simulink model "BuckConverter_Speed_first"  (R2021a)
settings: Solver=ode15s  StartTime=0.0  StopTime=0.01  MaxStep=1/(4*fsw)  RelTol=1e-3
PreLoadFcn:
  | Param_BuckConvertrer
undefined symbols (not defined in the file): DeadTime, fsw, MaxDuty, MinDuty, TimerCountMax
libraries: fl_lib x10, nesl_utility x6, ee_lib x2, eeGeneralControl x1, simulink x1
settings Model: Creator=ykamatan  LastModifiedBy=ykamatan
settings SimscapeCC: SimscapeLogType=local  SimscapeLogSimulationStatistics=on  SimscapeLogName=simlogBuckConverter  SimscapeLogLimitData=off

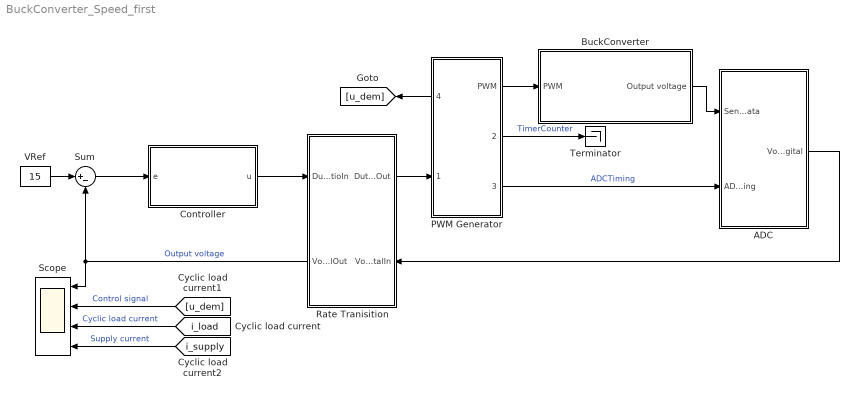
== system BuckConverter_Speed_first ==
  ADC : Subsystem
      settings: PortSchema="{\"entries\":[{\"content\":{\"sides\":[{\"content\":{\"connectorIds\":[]},\"type\":\"ConnectorPlacement.EquallySpacedRectSide\",\"uuid\":\"bf6494ef-7686-469c-b9a7-d936a514d7bb\"},{\"content\":{\"connectorIds\":[],\"side\":\"RIGHT\"},\"type\":\"ConnectorPlacement.EquallySpacedRectSide\",\"uuid\":\"0950a60e-c0cc-4272-a83f-094f77322897\"},{\"content\":{\"connectorIds\":[\"In1\",\"In2\"],\"side\":\"TOP\"},\"type\":\"ConnectorPlacement.EquallySpacedRectSide\",\"uuid\":\"00c09912-fdc2-48e7-8c4d-a5acc3c27a79\"},{\"content\":{\"connectorIds\":[\"Out1\"],\"side\":\"BOTTOM\"},\"type\":\"ConnectorPlacement.EquallySpacedRectSide\",\"uuid\":\"03f25cec-c069-475d-9cdb-f76905a62459\"}]},\"type\":\"ConnectorPlacement.EquallySpacedConnector\",\"uuid\":\"810e678a-0254-41ea-a955-7b792bb7817f\"}],\"packageUris\":[\"http://schema.mathworks.com/mf0/Connector/R2020b\"],\"version\":\"1.0\"}"
  BuckConverter : Subsystem
  Controller : Subsystem  Variant=on  VariantControlMode=label  LabelModeActiveChoice=Discrete
      settings: AttributesFormatString=%<BlockChoice>  PortSchema="{\"entries\":[{\"content\":{\"sides\":[{\"content\":{\"connectorIds\":[\"Out1\"]},\"type\":\"ConnectorPlacement.EquallySpacedRectSide\",\"uuid\":\"685b2dc6-4f02-4a7b-a6bf-88e3d36bc83e\"},{\"content\":{\"connectorIds\":[\"In1\"],\"side\":\"RIGHT\"},\"type\":\"ConnectorPlacement.EquallySpacedRectSide\",\"uuid\":\"22f020c9-8565-4c84-885b-1a26e9339655\"},{\"content\":{\"connectorIds\":[],\"side\":\"TOP\"},\"type\":\"ConnectorPlacement.EquallySpacedRectSide\",\"uuid\":\"adb99d42-7d64-4d3d-be76-0d683fbfb3ea\"}]},\"type\":\"ConnectorPlacement.EquallySpacedConnector\",\"uuid\":\"e1039069-23fc-4515-974b-2f79b4645018\"}],\"packageUris\":[\"http://schema.mathworks.com/mf0/Connector/R2020b\"],\"version\":\"1.0\"}"
  PWM Generator : Subsystem
      settings: PortSchema="{\"entries\":[{\"content\":{\"sides\":[{\"content\":{\"connectorIds\":[\"Out4\",\"In1\"]},\"type\":\"ConnectorPlacement.EquallySpacedRectSide\",\"uuid\":\"f1ce74a1-1a8f-47f7-9cd0-3fde2298587e\"},{\"content\":{\"connectorIds\":[\"Out1\",\"Out2\",\"Out3\"],\"side\":\"RIGHT\"},\"type\":\"ConnectorPlacement.EquallySpacedRectSide\",\"uuid\":\"07a21a0a-7c65-47ad-a570-3864e55861a7\"},{\"content\":{\"connectorIds\":[],\"side\":\"TOP\"},\"type\":\"ConnectorPlacement.EquallySpacedRectSide\",\"uuid\":\"8095ad0e-75cb-4fce-a461-a34c62050671\"},{\"content\":{\"connectorIds\":[],\"side\":\"BOTTOM\"},\"type\":\"ConnectorPlacement.EquallySpacedRectSide\",\"uuid\":\"dd227050-6090-4f15-8849-81744ca66faf\"}]},\"type\":\"ConnectorPlacement.EquallySpacedConnector\",\"uuid\":\"2f82d847-9a80-4fd2-b8a2-8a906b7e656c\"}],\"packageUris\":[\"http://schema.mathworks.com/mf0/Connector/R2020b\"],\"version\":\"1.0\"}"
  "Rate Tranisition " : Subsystem
      settings: PortSchema="{\"entries\":[{\"content\":{\"sides\":[{\"content\":{\"connectorIds\":[\"In1\",\"Out2\"]},\"type\":\"ConnectorPlacement.EquallySpacedRectSide\",\"uuid\":\"82fdd683-de0b-47f1-9418-2e57132da0d0\"},{\"content\":{\"connectorIds\":[\"Out1\",\"In2\"],\"side\":\"RIGHT\"},\"type\":\"ConnectorPlacement.EquallySpacedRectSide\",\"uuid\":\"07812756-bbdf-4a3e-b825-c2cce10242a3\"},{\"content\":{\"connectorIds\":[],\"side\":\"TOP\"},\"type\":\"ConnectorPlacement.EquallySpacedRectSide\",\"uuid\":\"2a69d2b0-ad53-492d-9041-fc24e9d8466e\"}]},\"type\":\"ConnectorPlacement.EquallySpacedConnector\",\"uuid\":\"5e8493d4-adb1-45a0-b631-53482b8c22b1\"}],\"packageUris\":[\"http://schema.mathworks.com/mf0/Connector/R2020b\"],\"version\":\"1.0\"}"
  Scope : Scope  NumInputPorts=4
  Sum : Sum  Inputs=|+-  InputSameDT=on  SaturateOnIntegerOverflow=on  OutDataTypeStr=Inherit: Same as first input
  Terminator : Terminator
  VRef : Constant  Value=15
  wires:
  Controller/1(u) -> "Rate Tranisition "/1(DutyRatioIn)
  Sum/1 -> Controller/1(e)
  VRef/1 -> Sum/1
  PWM Generator/3(TopDetect) -> ADC/2(ADCTiming)  "ADCTiming"
  [u_dem] -> Scope/2  "Control signal"
  [i_load] -> Scope/3  "Cyclic load current"
  [i_supply] -> Scope/4  "Supply current"
  ADC/1(Vo_Digital) -> "Rate Tranisition "/2(Vo_DigitalIn)
  "Rate Tranisition "/2(Vo_DigitalOut) -> Sum/2, Scope/1  "Output voltage"
  "Rate Tranisition "/1(DutyRatioOut) -> PWM Generator/1(DutyRatio)
  PWM Generator/4(DutyRatio_limited) -> [u_dem]
  PWM Generator/1(PWM) -> BuckConverter/1(PWM)
  BuckConverter/1(Output voltage) -> ADC/1(SensorData)
  PWM Generator/2(TimerCounter) -> Terminator/1  "TimerCounter"

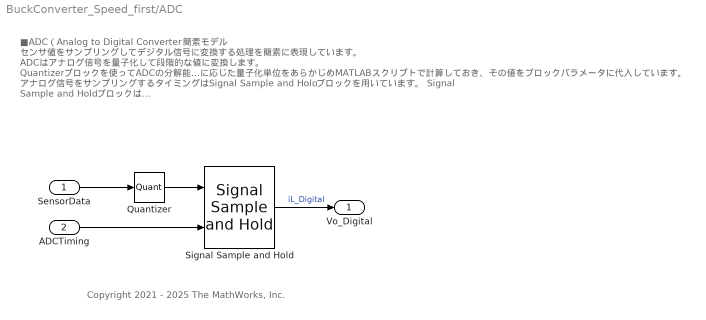
== system BuckConverter_Speed_first/ADC ==
  note: ■ADC（Analog to Digital Converter)簡素モデル
      | センサ値をサンプリングしてデジタル信号に変換する処理を簡素に表現しています。
      | ADCはアナログ信号を量子化して段階的な値に変換します。
      | Quantizerブロックを使ってADCの分解能に応じた量子化単位をあらかじめMATLABスクリプトで計算しておき、その値をブロックパラメータに代入しています。
      | アナログ信号をサンプリングするタイミングはSignal Sample and Holdブロックを用いています。
      | Signal Sample and Holdブロックは
      | Inにサンプリングしたい信号、Sにサンプリングタイミングを指定するパルス信号を入力することで、
      | そのタイミングでInの値をサンプリングし、それ以降次のパルスが入るまで値を保持します。
  note: Copyright 2021 - 2025 The MathWorks, Inc.
  SensorData : Inport
  ADCTiming : Inport  Port=2
  Quantizer : Quantizer  QuantizationInterval=QuantUnit
  Signal Sample and Hold : eeGeneralControl/Signal Sample and Hold  LabelModeActiveChoice=Discrete  x0=0  Ts=-1
      settings: SourceProductBaseCode=PS
  Vo_Digital : Outport
  wires:
  Quantizer/1 -> Signal Sample and Hold/1
  Signal Sample and Hold/1 -> Vo_Digital/1  "iL_Digital"
  ADCTiming/1 -> Signal Sample and Hold/2
  SensorData/1 -> Quantizer/1

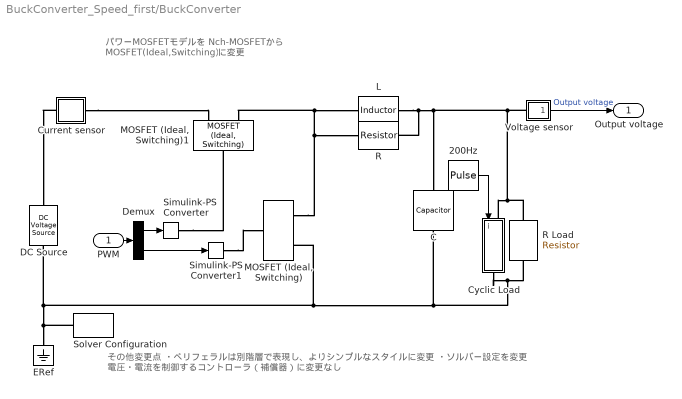
== system BuckConverter_Speed_first/BuckConverter ==
  note: その他変更点
      | ・ペリフェラルは別階層で表現し、よりシンプルなスタイルに変更
      | ・ソルバー設定を変更
      |
      | 電圧・電流を制御するコントローラ（補償器）に変更なし
  note: パワーMOSFETモデルを
      | Nch-MOSFETから
      | MOSFET(Ideal,Switching)に変更
  PWM : Inport
  " C" : fl_lib/Electrical/Electrical Elements/Capacitor  c=22 uF  r=0 Ohm  g=0 1/Ohm  i_specify=off  i_priority=High  i=0 A  i_nominal_specify=off  i_nominal_unit=A  i_nominal_value=1  v_specify=off  v_priority=High  v=0 V  v_nominal_specify=off  v_nominal_unit=V  v_nominal_value=1  vc_specify=on  vc_priority=High  vc=0 V  vc_nominal_specify=off  vc_nominal_unit=V  vc_nominal_value=1
  200Hz : DiscretePulseGenerator  PulseType=Time based  Period=1/200  PulseWidth=50  PhaseDelay=1/400
  Current sensor : Subsystem
  Cyclic Load : Subsystem
  DC Source : fl_lib/Electrical/Electrical Sources/DC Voltage Source  v0=30 V
      settings: AttributesFormatString=%<v0> %<v0_unit>
  Demux : Demux  Outputs=2
  ERef : fl_lib/Electrical/Electrical Elements/Electrical Reference
  L : fl_lib/Electrical/Electrical Elements/Inductor  l=1e-3 H  r=0 Ohm  g=0 1/Ohm  i_specify=off  i_priority=High  i=0 A  i_nominal_specify=off  i_nominal_unit=A  i_nominal_value=1  v_specify=off  v_priority=High  v=0 V  v_nominal_specify=off  v_nominal_unit=V  v_nominal_value=1  i_L_specify=on  i_L_priority=High  i_L=0 A  i_L_nominal_specify=off  i_L_nominal_unit=A  i_L_nominal_value=1
  "MOSFET (Ideal, Switching)" : ee_lib/Semiconductors & Converters/MOSFET (Ideal, Switching)  Rds=0.1 Ohm  Goff=1e-6 1/Ohm  Vth=2 V  diode_param=2  diode_Vf=0.8 V  diode_Ron=0.001 Ohm  diode_Goff=1e-5 1/Ohm  diode_C=50e-9 F  diode_iRM=-235 A  diode_iF=300 A  diode_idot=-50 A/us  diode_trr_param=1  diode_trr_factor=3  diode_trr=15 us  diode_Qrr=1500 s*uA  thermal_loss_option=ee.enum.converters.thermalLossOption.constantvalues  Von_data=[0, 1.1, 1.3, 1.45, 1.75, 2.25, 2.7; 0, 1, 1.15, 1.35, 1.7, 2.35, 3] V  Eon_data=[0, .29, 1.43, 2.86, 5.71, 13.14, 22.86; 0, .57, 2.63, 5.14, 10.29, 20.57, 30.29] * 1e-3 J  Eoff_data=[0, .21, 1.07, 2.14, 4.29, 9.86, 17.14; 0, .43, 1.97, 3.86, 7.71, 15.43, 22.71] * 1e-3 J  Tj=[298.15, 398.15] K  Iout_data=[0, 10, 50, 100, 200, 400, 600] A  Eon_scalar=22.86e-3 J  Eoff_scalar=17.14e-3 J  Voff=300 V  Iout_scalar=600 A  diodeModelType=ee.enum.converters.diodeModelType.pwl  diode_IfMat=[.07, .12, .19, 1.75, 4.24, 7.32, 11.2; .16, .3, .72, 2.14, 4.02, 6.35, 9.12] A  diode_TjVec=[25, 125] degC  diode_VfVec=[.5, .7, .9, 1.3, 1.7, 2.1, 2.5] V  thermal_network_parameterization=ee.enum.thermalNetworkTopology.external  Rth=[.03, .2] K/W  Rth_Foster=[.03, .2] K/W  thermal_mass_parameterization=ee.enum.thermalNetwork.timeconstant  thermal_mass=[3, 25] J/K  thermal_mass_Foster=[33, 50] J/K  thermal_time_constant=[.1, 5] s  thermal_time_constant_Foster=[1, 10] s  thermal_mass_initial_temperatures=[25, 25] degC  junction_thermal_mass=0.1 J/K  vT_specify=off  vT_priority=None  vT=0 V  vT_nominal_specify=off  vT_nominal_unit=V  vT_nominal_value=1  Qj_specify=off  Qj_priority=None  Qj=0 W  Qj_nominal_specify=off  Qj_nominal_unit=W  Qj_nominal_value=1  junction_temperature_specify=off  junction_temperature_priority=None  junction_temperature=25 degC  junction_temperature_nominal_specify=off  junction_temperature_nominal_unit=degC  junction_temperature_nominal_value=1
  "MOSFET (Ideal, Switching)1" : ee_lib/Semiconductors & Converters/MOSFET (Ideal, Switching)  Rds=0.1 Ohm  Goff=1e-6 1/Ohm  Vth=2 V  diode_param=2  diode_Vf=0.8 V  diode_Ron=0.001 Ohm  diode_Goff=1e-5 1/Ohm  diode_C=50e-9 F  diode_iRM=-235 A  diode_iF=300 A  diode_idot=-50 A/us  diode_trr_param=1  diode_trr_factor=3  diode_trr=15 us  diode_Qrr=1500 s*uA  thermal_loss_option=ee.enum.converters.thermalLossOption.constantvalues  Von_data=[0, 1.1, 1.3, 1.45, 1.75, 2.25, 2.7; 0, 1, 1.15, 1.35, 1.7, 2.35, 3] V  Eon_data=[0, .29, 1.43, 2.86, 5.71, 13.14, 22.86; 0, .57, 2.63, 5.14, 10.29, 20.57, 30.29] * 1e-3 J  Eoff_data=[0, .21, 1.07, 2.14, 4.29, 9.86, 17.14; 0, .43, 1.97, 3.86, 7.71, 15.43, 22.71] * 1e-3 J  Tj=[298.15, 398.15] K  Iout_data=[0, 10, 50, 100, 200, 400, 600] A  Eon_scalar=22.86e-3 J  Eoff_scalar=17.14e-3 J  Voff=300 V  Iout_scalar=600 A  diodeModelType=ee.enum.converters.diodeModelType.pwl  diode_IfMat=[.07, .12, .19, 1.75, 4.24, 7.32, 11.2; .16, .3, .72, 2.14, 4.02, 6.35, 9.12] A  diode_TjVec=[25, 125] degC  diode_VfVec=[.5, .7, .9, 1.3, 1.7, 2.1, 2.5] V  thermal_network_parameterization=ee.enum.thermalNetworkTopology.external  Rth=[.03, .2] K/W  Rth_Foster=[.03, .2] K/W  thermal_mass_parameterization=ee.enum.thermalNetwork.timeconstant  thermal_mass=[3, 25] J/K  thermal_mass_Foster=[33, 50] J/K  thermal_time_constant=[.1, 5] s  thermal_time_constant_Foster=[1, 10] s  thermal_mass_initial_temperatures=[25, 25] degC  junction_thermal_mass=0.1 J/K  vT_specify=off  vT_priority=None  vT=0 V  vT_nominal_specify=off  vT_nominal_unit=V  vT_nominal_value=1  Qj_specify=off  Qj_priority=None  Qj=0 W  Qj_nominal_specify=off  Qj_nominal_unit=W  Qj_nominal_value=1  junction_temperature_specify=off  junction_temperature_priority=None  junction_temperature=25 degC  junction_temperature_nominal_specify=off  junction_temperature_nominal_unit=degC  junction_temperature_nominal_value=1
  R : fl_lib/Electrical/Electrical Elements/Resistor  R=10 kOhm  i_specify=off  i_priority=High  i=0 A  i_nominal_specify=off  i_nominal_unit=A  i_nominal_value=1  v_specify=off  v_priority=High  v=0 V  v_nominal_specify=off  v_nominal_unit=V  v_nominal_value=1
  R Load : fl_lib/Electrical/Electrical Elements/Resistor  R=3.75 Ohm  i_specify=off  i_priority=High  i=0 A  i_nominal_specify=off  i_nominal_unit=A  i_nominal_value=1  v_specify=off  v_priority=High  v=0 V  v_nominal_specify=off  v_nominal_unit=V  v_nominal_value=1
  Simulink-PS Converter : nesl_utility/Simulink-PS Converter  PhysicalDomain=network_engine_domain  SubClassName=ps_input  LeftPortType=input  RightPortType=output  PseudoPeriodic=off  Frequencies=[]  NoiseDistribution=none  NoiseParameters=[]  Unit=1  AffineConversion=off  FilteringAndDerivatives=provide  SimscapeFilterOrder=1  InputFilterTimeConstant=0.001  UdotUserProvided=0
      settings: SourceProductBaseCode=PW,SS
  Simulink-PS Converter1 : nesl_utility/Simulink-PS Converter  PhysicalDomain=network_engine_domain  SubClassName=ps_input  LeftPortType=input  RightPortType=output  PseudoPeriodic=off  Frequencies=[]  NoiseDistribution=none  NoiseParameters=[]  Unit=1  AffineConversion=off  FilteringAndDerivatives=provide  SimscapeFilterOrder=1  InputFilterTimeConstant=0.001  UdotUserProvided=0
      settings: SourceProductBaseCode=PW,SS
  Solver Configuration : nesl_utility/Solver Configuration  PhysicalDomain=network_engine_domain  SubClassName=solver  LeftPortType=input  RightPortType=generic  Tones=[]  Harmonics=[]  SimulateNoise=off  Profile=off  UseLocalSampling=off  EnableSwitchedLinearOptims=on  FrequencyDomain=off  UseCCode=off  RelTol=0.001  AbsTol=1e-06  MinStep=1e-09  ToWorkspace=off  RevertToSquareIcSolve=off  NumHomotopyIterations=100  PhasorMode=off  PhasorModeNumHarmonics=1  DoDC=off  ResidualTolerance=1e-9  UseLocalSolver=off  LocalSolverChoice=NE_BACKWARD_EULER_ADVANCER  LocalSolverSampleTime=1e-7  DoFixedCost=off  MaxNonlinIter=12  MaxModeIter=2  ComputeImpulses=off  ImpulseIterations=1  LinearAlgebra=auto  EquationFormulation=NE_TIME_EF  DelaysMemoryBudget=1024  AutomaticFiltering=on  FilteringTimeConstant=0.001  PartitionStorageMethod=AS_NEEDED  PartitionMemoryBudget=1024  PartitionMethod=FAST
      settings: SourceProductBaseCode=PW,SS
  Voltage sensor : Subsystem
      settings: CopyFcn=set_param(gcb,'LinkStatus','none')
  Output voltage : Outport
  wires:
  Demux/1 -> Simulink-PS Converter/1
  Demux/2 -> Simulink-PS Converter1/1
  PWM/1 -> Demux/1
  200Hz/1 -> Cyclic Load/1(i)
  Voltage sensor/1(v) -> Output voltage/1  "Output voltage"
  connections:
  R Load/LConn1 -- Voltage sensor/LConn1 -- L/LConn1 -- R/LConn1 -- " C"/LConn1 -- Cyclic Load/LConn1
  "MOSFET (Ideal, Switching)"/RConn1 -- R/RConn1 -- L/RConn1 -- "MOSFET (Ideal, Switching)1"/RConn2
  " C"/RConn1 -- Cyclic Load/RConn1 -- R Load/RConn1 -- "MOSFET (Ideal, Switching)"/RConn2 -- DC Source/RConn1 -- Solver Configuration/RConn1 -- ERef/LConn1
  Current sensor/RConn1 -- "MOSFET (Ideal, Switching)1"/RConn1
  Current sensor/LConn1 -- DC Source/LConn1
  Simulink-PS Converter1/RConn1 -- "MOSFET (Ideal, Switching)"/LConn1
  Simulink-PS Converter/RConn1 -- "MOSFET (Ideal, Switching)1"/LConn1

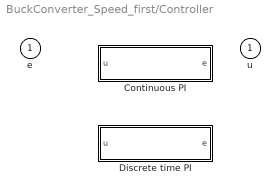
== system BuckConverter_Speed_first/Controller ==
  e : Inport
  Continuous PI : Subsystem  VariantControl=Continuous
  Discrete time PI : Subsystem  VariantControl=Discrete
  u : Outport  VectorParamsAs1DForOutWhenUnconnected=off

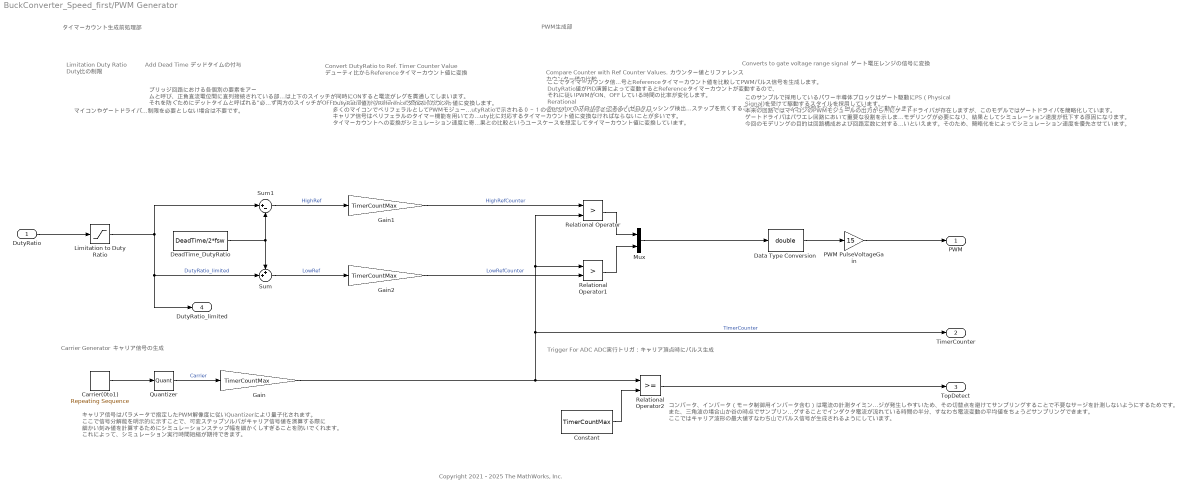
== system BuckConverter_Speed_first/PWM Generator ==
  note: PWM生成部
  note: タイマーカウント生成前処理部
  note: Limitation
      | Duty Ratio
      |
      | Duty比の制限
  note: キャリア信号はパラメータで指定したPWM解像度に従いQuantizerにより量子化されます。
      | ここで信号分解能を明示的に示すことで、可変ステップソルバがキャリア信号値を演算する際に
      | 細かい刻み値を計算するためにシミュレーションステップ幅を細かくしすぎることを防いでくれます。
      | これによって、シミュレーション実行時間短縮が期待できます。
  note: Converts to gate voltage range signal
      | ゲート電圧レンジの信号に変換
  note: Compare Counter with Ref Counter Values.
      | カウンター値とリファレンス カウンター値の比較
  note: Trigger For ADC
      | ADC実行トリガ：キャリア頂点時にパルス生成
  note: Convert DutyRatio to　Ref. Timer Counter Value
      | デューティ比からReferenceタイマーカウント値に変換
  note: Add Dead Time
      | デッドタイムの付与
  note: Carrier Generator
      | キャリア信号の生成
  note: Copyright 2021 - 2025 The MathWorks, Inc.
  note: ブリッジ回路における各個別の要素をアー ムと呼び、正負直流電位間に直列接続されている部分を上下一組でレグと呼びます。今回回路に用いているハーフブリッジ回路は単一のレグに相当します。レグを駆動する際には上下のスイッチが同時にONすると電流がレグを貫通してしまいます。
      | それを防ぐためにデットタイムと呼ばれる”必ず両方のスイッチがOFFとなる時間”を付与することで貫通を防ぎます。
  note: DutyRatio値からReferenceタイマーカウント値に変換します。
      | 多くのマイコンでペリフェラルとしてPWMモジュールが搭載されていますが、DutyRatioで示される０～１の値を使ってPWM波形を生成していません。
      |
      | キャリア信号はペリフェラルのタイマー機能を用いてカウントアップ・カウントダウンによって生成されるカウント値として指定されるので、Duty値もまた、Duty比に対応するタイマーカウント値に変換なければならないことが多いです。
      | タイマーカウントへの変換がシミュレーション速度に寄与する影響度は少ないですが、実機実験でのデバック結果との比較というユースケースを想定してタイマーカウント値に変換しています。
  note: ここでタイマーカウンタ信号とReferenceタイマーカウント値を比較してPWMパルス信号を生成します。
      |
      | DutyRatio値がPID演算によって変動するとReferenceタイマーカウントが変動するので、
      | それに従いPWMがON、OFFしている時間の比率が変化します。
      | Rerational Operatorのプロパティである「ゼロクロッシング検出を有効にする」を有効にすることで、可変ステップソルバは比較によって値が変動するタイミングで細かくステップを刻み、そうでない箇所ではタイムステップを荒くすることでシミュレーション時間をなるべく短くするように動作します。
  note: このサンプルで採用しているパワー半導体ブロックはゲート駆動にPS（Physical Signal)を受けて駆動するスタイルを採用しています。
      |
      | 本来の回路ではマイコンのPWMモジュールの出力からパワー半導体デバイスの間にゲートドライバが存在しますが、このモデルではゲートドライバを簡略化しています。
      |
      | ゲートドライバはパワエレ回路において重要な役割を示しますが、正確な挙動表現には細かいモデリングが必要になり、結果としてシミュレーション速度が低下する原因になります。
      | 今回のモデリングの目的は回路構成および回路定数に対する適切な制御則の導出であるため、目的に対してゲートドライバの詳細表現は影響度が少ないといえます。そのため、簡略化をによってシミュレーション速度を優先させています。
  note: コンバータ、インバータ（モータ制御用インバータ含む）は電流の計測タイミングをPWMキャリア信号と同期させることが多く、ノコギリ波の頂点、もしくは三角波の山か谷のタイミングでADCのサンプリングを行います。これはPWMパルス電圧が切り替わる瞬間は電流サージが発生しやすいため、その切替点を避けてサンプリングすることで不要なサージを計測しないようにするためです。
      | また、三角波の場合山か谷の時点でサンプリングすることでインダクタ電流が流れている時間の半分、すなわち電流変動の平均値をちょうどサンプリングできます。
      | ここではキャリア波形の最大値すなわち山でパルス信号が生成されるようにしています。
  note: マイコンやゲートドライバ、制御ICにはDutyの最大値、最小値が指定されているものも多いためここで制限を設けています。制限を必要としない場合は不要です。
  DutyRatio : Inport
  Carrier(0to1) : simulink/Sources/Repeating Sequence  rep_seq_t=[0 1/fsw/2 1/fsw]  rep_seq_y=[1 0 1]
  Constant : Constant  Value=TimerCountMax  OutDataTypeStr=uint16
  Data Type Conversion : DataTypeConversion  OutDataTypeStr=double
  DeadTime_DutyRatio : Constant  Value=DeadTime/2*fsw  OutDataTypeStr=double
  Gain : Gain  Gain=TimerCountMax  OutDataTypeStr=double
  Gain1 : Gain  Gain=TimerCountMax
  Gain2 : Gain  Gain=TimerCountMax  OutDataTypeStr=double
  Limitation to Duty Ratio : Saturate  UpperLimit=MaxDuty  LowerLimit=MinDuty
  Mux : Mux  Inputs=2
  PWM PulseVoltageGain : Gain  Gain=15
  Quantizer : Quantizer  QuantizationInterval=PWM_Resolution
  Relational Operator : RelationalOperator  Operator=>  OutDataTypeStr=boolean  RndMeth=Simplest  InputSameDT=on
  Relational Operator1 : RelationalOperator  Operator=>  OutDataTypeStr=boolean  RndMeth=Simplest  InputSameDT=on
  Relational Operator2 : RelationalOperator  OutDataTypeStr=boolean  RndMeth=Simplest
  Sum : Sum  Inputs=++|
  Sum1 : Sum  Inputs=|+-
  PWM : Outport
  TimerCounter : Outport  Port=2
  TopDetect : Outport  Port=3
  DutyRatio_limited : Outport  Port=4
  wires:
  Relational Operator1/1 -> Mux/2
  Data Type Conversion/1 -> PWM PulseVoltageGain/1
  Mux/1 -> Data Type Conversion/1
  Relational Operator/1 -> Mux/1
  DutyRatio/1 -> Limitation to Duty Ratio/1
  PWM PulseVoltageGain/1 -> PWM/1
  Carrier(0to1)/1 -> Quantizer/1
  Sum/1 -> Gain2/1  "LowRef"
  Limitation to Duty Ratio/1 -> DutyRatio_limited/1, Sum/2, Sum1/1  "DutyRatio_limited"
  DeadTime_DutyRatio/1 -> Sum1/2, Sum/1
  Constant/1 -> Relational Operator2/2
  Relational Operator2/1 -> TopDetect/1
  Quantizer/1 -> Gain/1  "Carrier"
  Gain/1 -> Relational Operator2/1, Relational Operator1/1, Relational Operator/2, TimerCounter/1  "TimerCounter"
  Gain1/1 -> Relational Operator/1  "HighRefCounter"
  Sum1/1 -> Gain1/1  "HighRef"
  Gain2/1 -> Relational Operator1/2  "LowRefCounter"

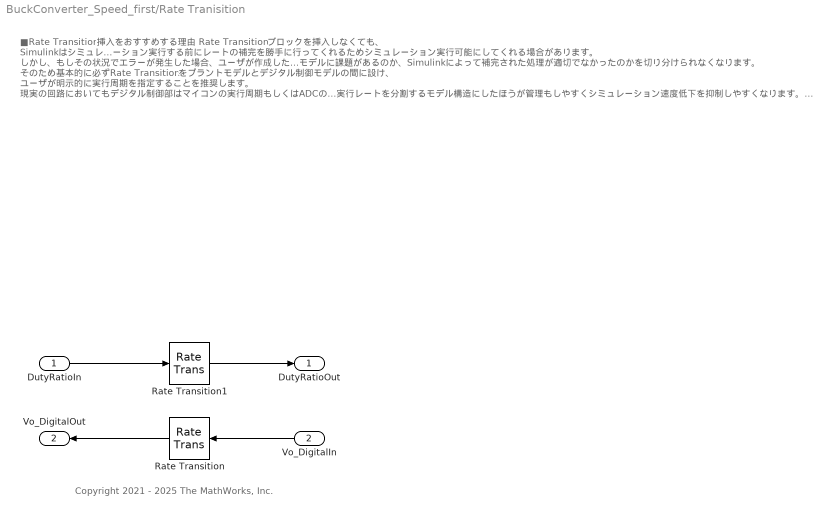
== system BuckConverter_Speed_first/Rate Tranisition  ==
  note: ■Rate Transition挿入をおすすめする理由
      | Rate Transitionブロックを挿入しなくても、
      | Simulinkはシミュレーション実行する前にレートの補完を勝手に行ってくれるためシミュレーション実行可能にしてくれる場合があります。
      |
      | しかし、もしその状況でエラーが発生した場合、ユーザが作成したモデルに課題があるのか、Simulinkによって補完された処理が適切でなかったのかを切り分けられなくなります。
      |
      | そのため基本的に必ずRate Transitionをプラントモデルとデジタル制御モデルの間に設け、
      | ユーザが明示的に実行周期を指定することを推奨します。
      |
      | 現実の回路においてもデジタル制御部はマイコンの実行周期もしくはADCの変換タイミングをトリガーに周期的に処理を行うため、明示的に実行レートを分割するモデル構造にしたほうが管理もしやすくシミュレーション速度低下を抑制しやすくなります。
      |
      | ■Rate Transitionのブロックパラメータ設定方法
      | ・データ転送中の整合性を確保
      | ・確定的にデータ転送を確保（最大遅延）
      | のチェックを入れておくことで、想定される最大のサンプリング遅れでサンプル値を取得するようにシミュレーションが動作します。これにより代数ループ警告も回避することができます。
      | ただし、このモデルのサンプリングはデジタルControllerモデルの実行周期(Tcnt = 1/fsw）分だけ必ずサンプリング値が遅れて伝搬されるため、制御ループの伝達関数を解析した際のむだ時間遅れは常に最悪の e^-sTcntとなることに注意が必要です。
  note: Copyright 2021 - 2025 The MathWorks, Inc.
  DutyRatioIn : Inport
  Vo_DigitalIn : Inport  Port=2
  Rate Transition : RateTransition  OutPortSampleTime=1/fsw
  Rate Transition1 : RateTransition  InitialCondition=0.5
  DutyRatioOut : Outport
  Vo_DigitalOut : Outport  Port=2
  wires:
  Rate Transition/1 -> Vo_DigitalOut/1
  DutyRatioIn/1 -> Rate Transition1/1
  Rate Transition1/1 -> DutyRatioOut/1
  Vo_DigitalIn/1 -> Rate Transition/1

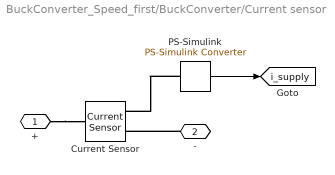
== system BuckConverter_Speed_first/BuckConverter/Current sensor ==
  Current Sensor : fl_lib/Electrical/Electrical Sensors/Current Sensor
  PS-Simulink : nesl_utility/PS-Simulink Converter  PhysicalDomain=network_engine_domain  SubClassName=ps_output  LeftPortType=input  RightPortType=output  PseudoPeriodic=off  Frequencies=[]  Unit=A  AffineConversion=off
      settings: SourceProductBaseCode=PW,SS
  + : PMIOPort  Side=Left
  - : PMIOPort  Port=2  Side=Right
  tag scope: i_supply=global
  wires:
  PS-Simulink/1 -> [i_supply]
  connections:
  PS-Simulink/LConn1 -- Current Sensor/RConn1
  +/RConn1 -- Current Sensor/LConn1
  -/RConn1 -- Current Sensor/RConn2

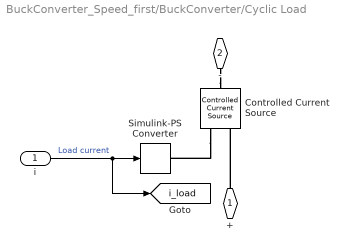
== system BuckConverter_Speed_first/BuckConverter/Cyclic Load ==
  i : Inport
  Controlled Current Source : fl_lib/Electrical/Electrical Sources/Controlled Current Source
  Simulink-PS Converter : nesl_utility/Simulink-PS Converter  PhysicalDomain=network_engine_domain  SubClassName=ps_input  LeftPortType=input  RightPortType=output  PseudoPeriodic=off  Frequencies=[]  NoiseDistribution=none  NoiseParameters=[]  Unit=A  AffineConversion=off  FilteringAndDerivatives=zero  SimscapeFilterOrder=1  InputFilterTimeConstant=.001  UdotUserProvided=0
      settings: SourceProductBaseCode=PW,SS
  + : PMIOPort  Side=Left
  - : PMIOPort  Port=2  Side=Right
  tag scope: i_load=global
  wires:
  i/1 -> Simulink-PS Converter/1, [i_load]  "Load current"
  connections:
  Controlled Current Source/RConn1 -- Simulink-PS Converter/RConn1
  +/RConn1 -- Controlled Current Source/RConn2
  -/RConn1 -- Controlled Current Source/LConn1

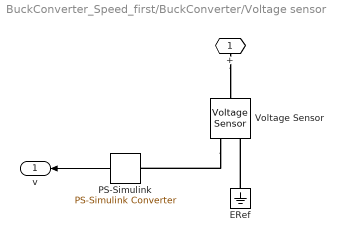
== system BuckConverter_Speed_first/BuckConverter/Voltage sensor ==
  ERef : fl_lib/Electrical/Electrical Elements/Electrical Reference
  PS-Simulink : nesl_utility/PS-Simulink Converter  PhysicalDomain=network_engine_domain  SubClassName=ps_output  LeftPortType=input  RightPortType=output  PseudoPeriodic=off  Frequencies=[]  Unit=V  AffineConversion=off
      settings: SourceProductBaseCode=PW,SS
  Voltage Sensor : fl_lib/Electrical/Electrical Sensors/Voltage Sensor
  + : PMIOPort  Side=Left
  v : Outport  VectorParamsAs1DForOutWhenUnconnected=off
  wires:
  PS-Simulink/1 -> v/1
  connections:
  Voltage Sensor/RConn1 -- PS-Simulink/LConn1
  +/RConn1 -- Voltage Sensor/LConn1
  ERef/LConn1 -- Voltage Sensor/RConn2

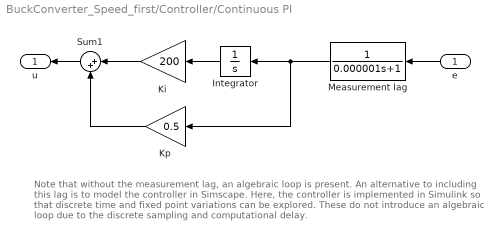
== system BuckConverter_Speed_first/Controller/Continuous PI ==
  note: Note that without the measurement lag, an algebraic loop is present. An alternative to
      | including this lag is to model the controller in Simscape. Here, the controller is implemented
      | in Simulink so that discrete time and fixed point variations can be explored. These do not
      | introduce an algebraic loop due to the discrete sampling and computational delay.
  e : Inport
  Integrator : Integrator
  Ki : Gain  Gain=200
  Kp : Gain  Gain=0.5
  Measurement lag : TransferFcn  Denominator=[0.000001 1]
  Sum1 : Sum  Inputs=|++  InputSameDT=on  SaturateOnIntegerOverflow=on  OutDataTypeStr=Inherit: Same as first input
  u : Outport  VectorParamsAs1DForOutWhenUnconnected=off
  wires:
  Measurement lag/1 -> Integrator/1, Kp/1
  Ki/1 -> Sum1/1
  Sum1/1 -> u/1
  Kp/1 -> Sum1/2
  Integrator/1 -> Ki/1
  e/1 -> Measurement lag/1

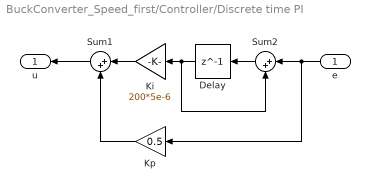
== system BuckConverter_Speed_first/Controller/Discrete time PI ==
  e : Inport
  Delay : Delay  DelayLength=1  SampleTime=5e-6
  Ki : Gain  Gain=200*5e-6
  Kp : Gain  Gain=0.5
  Sum1 : Sum  Inputs=|++  InputSameDT=on  SaturateOnIntegerOverflow=on  OutDataTypeStr=Inherit: Same as first input
  Sum2 : Sum  Inputs=|++  InputSameDT=on  SaturateOnIntegerOverflow=on  OutDataTypeStr=Inherit: Same as first input
  u : Outport  VectorParamsAs1DForOutWhenUnconnected=off
  wires:
  Ki/1 -> Sum1/1
  Sum2/1 -> Delay/1
  Delay/1 -> Ki/1, Sum2/2
  Kp/1 -> Sum1/2
  e/1 -> Sum2/1, Kp/1
  Sum1/1 -> u/1
